simulink library "constantBasisParameters_cl"  (R2018b)
settings: Solver=VariableStepAuto  StartTime=0.0  StopTime=10.0  RelTol=1e-3
undefined symbols (not defined in the file or in its folder): initializeBussesFromBlock
settings Model: Creator=mcobb  LastModifiedBy=mcobb

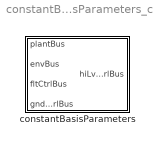
== system constantBasisParameters_cl ==
  constantBasisParameters : Subsystem  LoadFcn=initializeBussesFromBlock(gcb)  InitFcn=initializeBussesFromBlock(gcb)  StartFcn=initializeBussesFromBlock(gcb)  mask{basisParams=[1 1 1]}
      mask prompts: basisParams "Basis Parameters"

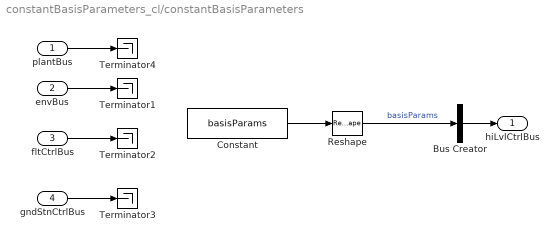
== system constantBasisParameters_cl/constantBasisParameters ==
  plantBus : Inport  OutDataTypeStr=Bus: plantBus
  envBus : Inport  Port=2  OutDataTypeStr=Bus: envBus
  fltCtrlBus : Inport  Port=3  OutDataTypeStr=Bus: fltCtrlBus
  gndStnCtrlBus : Inport  Port=4  OutDataTypeStr=Bus: gndStnCtrlBus
  Bus Creator : BusCreator  Inputs=1  OutDataTypeStr=Bus: hiLvlCtrlBus
  Constant : Constant  Value=basisParams
  Reshape : Reshape  OutputDimensionality=Column vector (2-D)
  Terminator{1..4} (4 alike) : Terminator
  hiLvlCtrlBus : Outport  OutDataTypeStr=Bus: hiLvlCtrlBus
  wires:
  envBus/1 -> Terminator1/1
  gndStnCtrlBus/1 -> Terminator3/1
  Bus Creator/1 -> hiLvlCtrlBus/1
  Constant/1 -> Reshape/1
  fltCtrlBus/1 -> Terminator2/1
  plantBus/1 -> Terminator4/1
  Reshape/1 -> Bus Creator/1  "basisParams"
